simulink model "ContinuousExample"  (R2015a)
settings: Solver=ode45  StartTime=0.0  StopTime=10.0  MaxStep=0.1  RelTol=1e-3
settings Model: Creator=jkapinski  LastModifiedBy=alex
settings DataIOCC: SaveFinalState=on  SaveFormat=StructureWithTime  SignalLoggingSaveFormat=ModelDataLogs
settings OptimizationCC: ExpressionDepthLimit=2147483647
settings DebuggingCC: UnderspecifiedInitializationDetection=Classic  MergeDetectMultiDrivingBlocksExec=none  SolverPrmCheckMsg=warning  MultiTaskDSMMsg=warning  MultiTaskCondExecSysMsg=none  FcnCallInpInsideContextMsg=UseLocalSettings  StateNameClashWarn=warning  InitInArrayFormatMsg=none
settings GRTTargetCC: CombineOutputUpdateFcns=off  GRTInterface=on

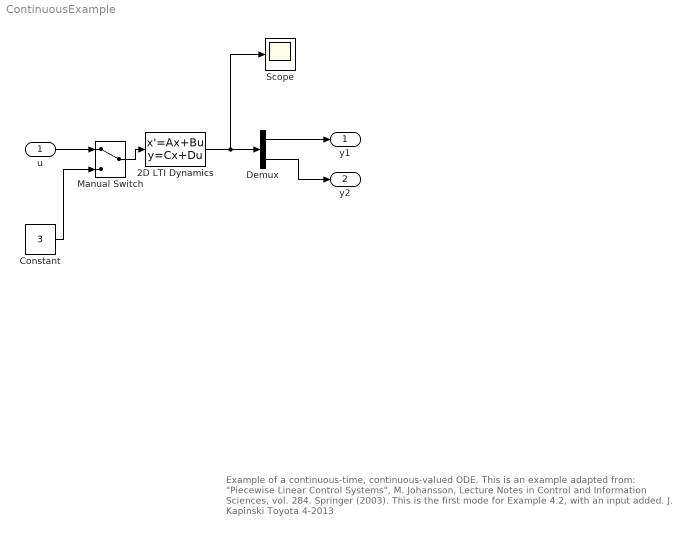
== system ContinuousExample ==
  note: Example of a continuous-time, continuous-valued ODE.
      | This is an example adapted from:
      | "Piecewise Linear Control Systems", M. Johansson, Lecture Notes in
      | Control and Information Sciences, vol. 284. Springer (2003).
      | This is the first mode for Example 4.2, with an input added.
      |
      | J. Kapinski
      | Toyota
      | 4-2013
  u : Inport
  2D LTI Dynamics : StateSpace  A=[-0.1 1.0;-10.0 -0.1]  B=[1.0;1.0]  C=eye(2)  D=[0;0]  X0=[1;1]
  Constant : Constant  Value=3
  Demux : Demux  Outputs=2
  Manual Switch : ManualSwitch
  Scope : Scope
  y1 : Outport
  y2 : Outport  Port=2
  wires:
  2D LTI Dynamics/1 -> Scope/1, Demux/1
  Demux/1 -> y1/1
  Demux/2 -> y2/1
  Constant/1 -> Manual Switch/2
  Manual Switch/1 -> 2D LTI Dynamics/1
  u/1 -> Manual Switch/1
